simulink model "passiveSuspension"  (R2024a)
settings: Solver=ode4  StartTime=0.0  StopTime=10  FixedStep=Ts  RelTol=1e-3
values from neighbouring files (symbols this model uses):
  bs = 7.5    [initparams.m]
  bus = 5    [initparams.m]
  ks = 900    [initparams.m]
  kus = kt    (= 2500)    [initparams.m]
  ms = 2.45    [initparams.m]
  mus = mu    (= 1)    [initparams.m]
  Ts = 0.01    [initparams.m]
  z1_dot_init = 0    [initparams.m]
  z1_init = 0.005    [initparams.m]
  z2_dot_init = 0    [initparams.m]
  z2_init = 0    [initparams.m]
settings Model: Creator=aidan  LastModifiedBy=aidan
settings DebuggingCC: UnderSpecifiedDimensionMsg=warning

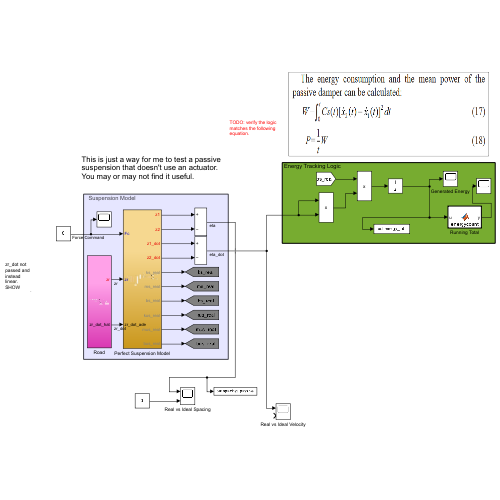
[thumbnail: Simulink's stored preview of the top-level diagram]
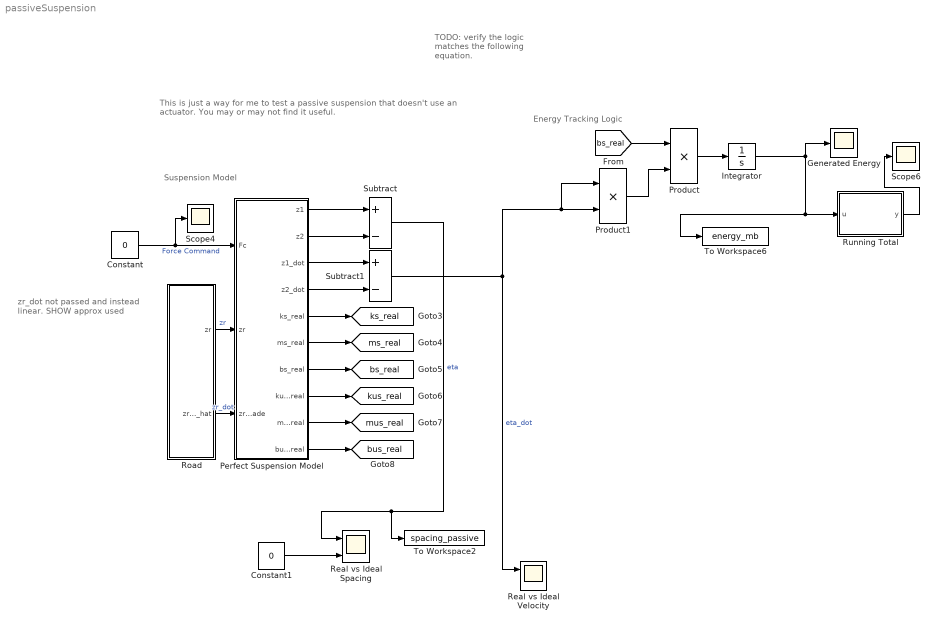
== system passiveSuspension ==
  note: This is just a way for me to test a passive suspension that doesn't use an actuator. You may or may not find it useful.
  note: zr_dot not passed and instead linear. SHOW approx used
  note: Suspension Model
  note: TODO: verify the logic matches the following equation.
  note: Energy Tracking Logic
  Constant : Constant  Value=0
  Constant1 : Constant  Value=0
  Generated Energy : Scope
  Integrator : Integrator
  Perfect Suspension Model : Subsystem
  Product : Product
  Product1 : Product
  Real vs Ideal Spacing : Scope  NumInputPorts=2
  Real vs Ideal Velocity : Scope  NumInputPorts=2
  Road : Subsystem
  Running Total : MATLAB Function  TreatAsAtomicUnit=on
  Scope4 : Scope
  Scope6 : Scope
  Subtract : Sum  Inputs=+-
  Subtract1 : Sum  Inputs=+-
  To Workspace2 : ToWorkspace  VariableName=spacing_passive  SaveFormat=Timeseries  SampleTime=-1
  To Workspace6 : ToWorkspace  VariableName=energy_mb  SaveFormat=Timeseries  SampleTime=-1
  tag scope: bs_real=global, bus_real=global, ks_real=global, kus_real=global, ms_real=global, mus_real=global
  wires:
  Perfect Suspension Model/5(ks_real) -> [ks_real]
  Perfect Suspension Model/6(ms_real) -> [ms_real]
  Perfect Suspension Model/7(bs_real) -> [bs_real]
  Perfect Suspension Model/8(kus_real) -> [kus_real]
  Perfect Suspension Model/9(mus_real) -> [mus_real]
  Perfect Suspension Model/10(bus_real) -> [bus_real]
  Perfect Suspension Model/3(z1_dot) -> Subtract1/1
  Perfect Suspension Model/4(z2_dot) -> Subtract1/2
  Perfect Suspension Model/2(z2) -> Subtract/2
  Subtract1/1 -> Real vs Ideal Velocity/1, Product1/2, Product1/1  "eta_dot"
  Constant/1 -> Perfect Suspension Model/1(Fc), Scope4/1  "Force Command"
  Subtract/1 -> Real vs Ideal Spacing/1, To Workspace2/1  "eta"
  Constant1/1 -> Real vs Ideal Spacing/2
  Perfect Suspension Model/1(z1) -> Subtract/1
  Running Total/1(y) -> Scope6/1
  Product/1 -> Integrator/1
  Integrator/1 -> Running Total/1(u), To Workspace6/1, Generated Energy/1
  [bs_real] -> Product/1
  Product1/1 -> Product/2
  Road/1(zr) -> Perfect Suspension Model/2(zr)  "zr"
  Road/2(zr_dot_hat) -> Perfect Suspension Model/3(zr_dot_ade)  "zr_dot"

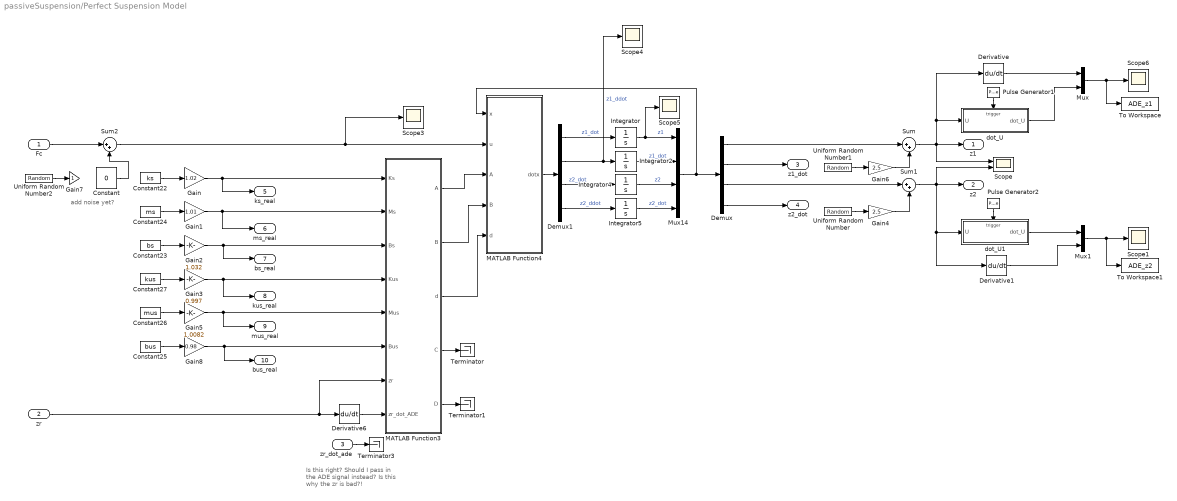
== system passiveSuspension/Perfect Suspension Model ==
  note: Is this right? Should I pass in the ADE signal instead? Is this why the zr is bad?!
  note: add noise yet?
  Fc : Inport
  zr : Inport  Port=2
  zr_dot_ade : Inport  Port=3
  Constant : Constant  Value=0
  Constant22 : Constant  Value=ks
  Constant23 : Constant  Value=bs
  Constant24 : Constant  Value=ms
  Constant25 : Constant  Value=bus
  Constant26 : Constant  Value=mus
  Constant27 : Constant  Value=kus
  Demux : Demux
  Demux1 : Demux
  Derivative : Derivative
  Derivative1 : Derivative
  Derivative6 : Derivative
  Gain : Gain  Gain=1.02
  Gain1 : Gain  Gain=1.01
  Gain2 : Gain  Gain=1.032
  Gain3 : Gain  Gain=0.997
  Gain4 : Gain  Gain=2.5
  Gain5 : Gain  Gain=1.0082
  Gain6 : Gain  Gain=2.5
  Gain7 : Gain
  Gain8 : Gain  Gain=0.98
  Integrator : Integrator  InitialCondition=z1_init
  Integrator2 : Integrator  InitialCondition=z1_dot_init
  Integrator4 : Integrator  InitialCondition=z2_init
  Integrator5 : Integrator  InitialCondition=z2_dot_init
  MATLAB Function3 : MATLAB Function  TreatAsAtomicUnit=on
  MATLAB Function4 : MATLAB Function  TreatAsAtomicUnit=on
  Mux : Mux  Inputs=2
  Mux1 : Mux  Inputs=2
  Mux14 : Mux
  Pulse Generator1 : DiscretePulseGenerator  PulseType=Time based  Period=Ts*2  PulseWidth=50
  Pulse Generator2 : DiscretePulseGenerator  PulseType=Time based  Period=Ts*2  PulseWidth=50
  Scope : Scope  NumInputPorts=2
  Scope{1,3..6} (5 alike) : Scope
  Sum : Sum  Inputs=|++
  Sum1 : Sum  Inputs=|++
  Sum2 : Sum  Inputs=|++
  Terminator : Terminator
  Terminator1 : Terminator
  Terminator3 : Terminator
  To Workspace : ToWorkspace  VariableName=ADE_z1  SampleTime=-1
  To Workspace1 : ToWorkspace  VariableName=ADE_z2  SampleTime=-1
  Uniform Random Number : UniformRandomNumber  Minimum=-1e-6  Maximum=1e-6  Seed=244334  SampleTime=Ts
  Uniform Random Number1 : UniformRandomNumber  Minimum=-1e-6  Maximum=1e-6  Seed=7  SampleTime=Ts
  Uniform Random Number2 : UniformRandomNumber  Minimum=-5e-3  Maximum=5e-3  Seed=89757  SampleTime=Ts
  dot_U : Subsystem  TreatAsAtomicUnit=on
  dot_U1 : Subsystem  TreatAsAtomicUnit=on
  z1 : Outport
  z2 : Outport  Port=2
  z1_dot : Outport  Port=3
  z2_dot : Outport  Port=4
  ks_real : Outport  Port=5
  ms_real : Outport  Port=6
  bs_real : Outport  Port=7
  kus_real : Outport  Port=8
  mus_real : Outport  Port=9
  bus_real : Outport  Port=10
  wires:
  Constant23/1 -> Gain2/1
  MATLAB Function3/4(C) -> Terminator/1
  Demux1/1 -> Integrator/1  "z1_dot"
  zr/1 -> MATLAB Function3/7(zr), Derivative6/1
  Integrator5/1 -> Mux14/4  "z2_dot"
  Demux1/2 -> Scope4/1, Integrator2/1  "z1_ddot"
  Gain2/1 -> bs_real/1, MATLAB Function3/3(Bs)
  Constant27/1 -> Gain3/1
  Gain3/1 -> kus_real/1, MATLAB Function3/4(Kus)
  Constant24/1 -> Gain1/1
  Constant25/1 -> Gain8/1
  Demux1/4 -> Integrator5/1  "z2_ddot"
  MATLAB Function4/1(dotx) -> Demux1/1
  Integrator4/1 -> Mux14/3  "z2"
  Integrator/1 -> Scope5/1, Mux14/1  "z1"
  Constant26/1 -> Gain5/1
  Gain8/1 -> bus_real/1, MATLAB Function3/6(Bus)
  MATLAB Function3/2(B) -> MATLAB Function4/4(B)
  Constant22/1 -> Gain/1
  Demux1/3 -> Integrator4/1  "z2_dot"
  Gain5/1 -> mus_real/1, MATLAB Function3/5(Mus)
  MATLAB Function3/5(D) -> Terminator1/1
  Integrator2/1 -> Mux14/2  "z1_dot"
  Gain1/1 -> ms_real/1, MATLAB Function3/2(Ms)
  Gain/1 -> ks_real/1, MATLAB Function3/1(Ks)
  MATLAB Function3/1(A) -> MATLAB Function4/3(A)
  Mux14/1 -> Demux/1, MATLAB Function4/1(x)
  MATLAB Function3/3(d) -> MATLAB Function4/5(d)
  Demux/2 -> z1_dot/1
  Demux/4 -> z2_dot/1
  Gain4/1 -> Sum1/2
  Uniform Random Number/1 -> Gain4/1
  Sum/1 -> Scope/1, Derivative/1, dot_U/1(U), z1/1
  Demux/1 -> Sum/1
  Demux/3 -> Sum1/1
  Uniform Random Number1/1 -> Gain6/1
  Gain6/1 -> Sum/2
  dot_U/1(dot_U) -> Mux/2
  Pulse Generator1/1 -> dot_U/Trigger
  Derivative/1 -> Mux/1
  Pulse Generator2/1 -> dot_U1/Trigger
  Sum1/1 -> Scope/2, Derivative1/1, dot_U1/1(U), z2/1
  dot_U1/1(dot_U) -> Mux1/1
  Derivative1/1 -> Mux1/2
  Sum2/1 -> Scope3/1, MATLAB Function4/2(u)
  Fc/1 -> Sum2/1
  Uniform Random Number2/1 -> Gain7/1
  Mux/1 -> To Workspace/1, Scope6/1
  Mux1/1 -> Scope1/1, To Workspace1/1
  Constant/1 -> Sum2/2
  zr_dot_ade/1 -> Terminator3/1
  Derivative6/1 -> MATLAB Function3/8(zr_dot_ADE)

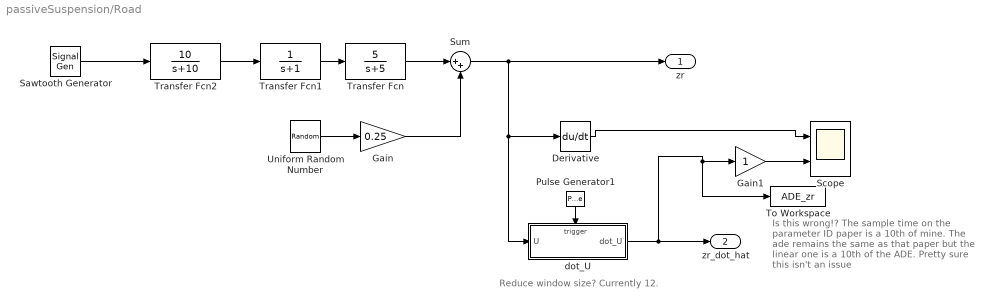
== system passiveSuspension/Road ==
  note: Is this wrong!? The sample time on the parameter ID paper is a 10th of mine. The ade remains the same as that paper but the linear one is a 10th of the ADE. Pretty sure this isn't an issue
  note: Reduce window size? Currently 12.
  Derivative : Derivative
  Gain : Gain  Gain=0.25
  Gain1 : Gain
  Pulse Generator1 : DiscretePulseGenerator  PulseType=Time based  Period=Ts*2  PulseWidth=50
  Sawtooth Generator : SignalGenerator  WaveForm=sawtooth  Amplitude=3.5e-2
  Scope : Scope  NumInputPorts=2
  Sum : Sum  Inputs=|++
  To Workspace : ToWorkspace  VariableName=ADE_zr  SampleTime=-1
  Transfer Fcn : TransferFcn  Numerator=[5]  Denominator=[1 5]
  Transfer Fcn1 : TransferFcn  Denominator=[1 1]
  Transfer Fcn2 : TransferFcn  Numerator=[10]  Denominator=[1 10]
  Uniform Random Number : UniformRandomNumber  Minimum=-1e-6  Maximum=1e-6  Seed=122334  SampleTime=Ts
  dot_U : Subsystem  TreatAsAtomicUnit=on
  zr : Outport
  zr_dot_hat : Outport  Port=2
  wires:
  Transfer Fcn2/1 -> Transfer Fcn1/1
  Transfer Fcn/1 -> Sum/1
  Sawtooth Generator/1 -> Transfer Fcn2/1
  Transfer Fcn1/1 -> Transfer Fcn/1
  Uniform Random Number/1 -> Gain/1
  Gain/1 -> Sum/2
  Sum/1 -> dot_U/1(U), Derivative/1, zr/1
  Pulse Generator1/1 -> dot_U/Trigger
  Derivative/1 -> Scope/1
  dot_U/1(dot_U) -> To Workspace/1, Gain1/1, zr_dot_hat/1
  Gain1/1 -> Scope/2

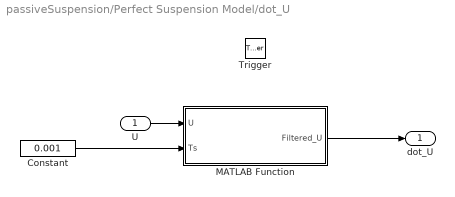
== system passiveSuspension/Perfect Suspension Model/dot_U ==
  U : Inport
  Trigger : TriggerPort  TriggerType=either  VariantControl=Variant  ZeroCross=off  PortDimensions=1
  Constant : Constant  Value=0.001
  MATLAB Function : MATLAB Function  TreatAsAtomicUnit=on
  dot_U : Outport  VectorParamsAs1DForOutWhenUnconnected=off
  wires:
  Constant/1 -> MATLAB Function/2(Ts)
  MATLAB Function/1(Filtered_U) -> dot_U/1
  U/1 -> MATLAB Function/1(U)

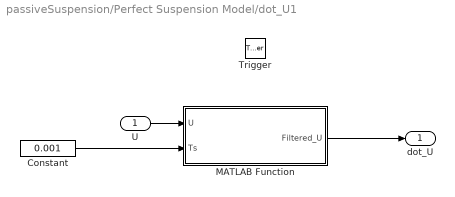
== system passiveSuspension/Perfect Suspension Model/dot_U1 ==
  U : Inport
  Trigger : TriggerPort  TriggerType=either  VariantControl=Variant  ZeroCross=off  PortDimensions=1
  Constant : Constant  Value=0.001
  MATLAB Function : MATLAB Function  TreatAsAtomicUnit=on
  dot_U : Outport  VectorParamsAs1DForOutWhenUnconnected=off
  wires:
  U/1 -> MATLAB Function/1(U)
  MATLAB Function/1(Filtered_U) -> dot_U/1
  Constant/1 -> MATLAB Function/2(Ts)

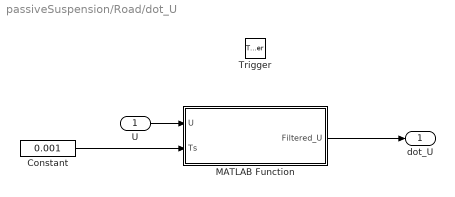
== system passiveSuspension/Road/dot_U ==
  U : Inport
  Trigger : TriggerPort  TriggerType=either  VariantControl=Variant  ZeroCross=off  PortDimensions=1
  Constant : Constant  Value=0.001
  MATLAB Function : MATLAB Function  TreatAsAtomicUnit=on
  dot_U : Outport  VectorParamsAs1DForOutWhenUnconnected=off
  wires:
  Constant/1 -> MATLAB Function/2(Ts)
  MATLAB Function/1(Filtered_U) -> dot_U/1
  U/1 -> MATLAB Function/1(U)

== matlab function passiveSuspension/Perfect Suspension Model/MATLAB Function3 ==
  data: Ks input; A output; Ms input; Bs input; Kus input; Mus input; Bus input; zr input; zr_dot_ADE input; B output; d output; C output; D output
function [A, B, d, C, D] = Syst(Ks, Ms, Bs, Kus, Mus, Bus, zr, zr_dot_ADE)
    A = [    0,      1,             0,              0; 
        -Ks/Ms, -Bs/Ms,         Ks/Ms,          Bs/Ms; 
             0,      0,             0,              1; 
        Ks/Mus, Bs/Mus, -(Kus+Ks)/Mus, -(Bus+Bs)/Mus];
 
    
    B = [0; 1/Ms; 0; -1/Mus];
    
    
    d = [0;    0; 0;  Kus/Mus*zr + Bus/Mus*zr_dot_ADE];
   
    
    C = [    1,      0,    -1,     0;
        -Ks/Ms, -Bs/Ms, Ks/Ms, Bs/Ms];
    
    D = [0; 1/Ms];
    
    
end

== matlab function passiveSuspension/Road/dot_U/MATLAB Function ==
  data: U input; Filtered_U output; Ts input
function Filtered_U = buffer(U,Ts)
    N = 12;
    %Ts = 0.001;
    persistent y;
    if isempty(y)
        y=zeros(N+1,1);
    end

    y = [U;y(1:end-1)];
    T = Ts*N;
    P = zeros(1,N+1);
    P_alpha = P;
    for k = 1:N+1
        tao_k = (k-1)*Ts;
        P(k) = T-2*tao_k;
        if((k==1)||(k==N+1))
            P_alpha(k) = P(k)*Ts/2;
        else
            P_alpha(k) = P(k)*Ts;
        end
    end
    
    Filtered_U = P_alpha*y*6/(T^3);

end

== matlab function passiveSuspension/Perfect Suspension Model/dot_U/MATLAB Function ==
  data: U input; Filtered_U output; Ts input
function Filtered_U = buffer(U,Ts)
    N = 10;
    %Ts = 0.001;
    persistent y;
    if isempty(y)
        y=zeros(N+1,1);
    end

    y = [U;y(1:end-1)];
    T = Ts*N;
    P = zeros(1,N+1);
    P_alpha = P;
    for k = 1:N+1
        tao_k = (k-1)*Ts;
        P(k) = T-2*tao_k;
        if((k==1)||(k==N+1))
            P_alpha(k) = P(k)*Ts/2;
        else
            P_alpha(k) = P(k)*Ts;
        end
    end
    
    Filtered_U = P_alpha*y*6/(T^3);

end

== matlab function passiveSuspension/Perfect Suspension Model/dot_U1/MATLAB Function ==
  data: U input; Filtered_U output; Ts input
function Filtered_U = buffer(U,Ts)
    N = 10;
    %Ts = 0.001;
    persistent y;
    if isempty(y)
        y=zeros(N+1,1);
    end

    y = [U;y(1:end-1)];
    T = Ts*N;
    P = zeros(1,N+1);
    P_alpha = P;
    for k = 1:N+1
        tao_k = (k-1)*Ts;
        P(k) = T-2*tao_k;
        if((k==1)||(k==N+1))
            P_alpha(k) = P(k)*Ts/2;
        else
            P_alpha(k) = P(k)*Ts;
        end
    end
    
    Filtered_U = P_alpha*y*6/(T^3);

end

== matlab function passiveSuspension/Running Total ==
  settings: updateMethod=DISCRETE
  data: u input; y output
function y = energycount(u)

persistent s;
if isempty(s)
    s = 0;
end
s = s + u;
y = s;

== matlab function passiveSuspension/Perfect Suspension Model/MATLAB Function4 ==
  data: x input; dotx output; u input; A input; B input; d input
function dotx  = Susp_System(x, u, A, B, d)
    
    dotx = A*x + B*u + d;
    %y = C*x + D*u;
end
